simulink model "Uebung5_A1_Anschauungsbeispiel"  (R2016a)
settings: Solver=VariableStepAuto  StartTime=0.0  StopTime=200000  RelTol=1e-3
undefined symbols (not defined in the file or in its folder): m, n
settings Model: Creator=gome  LastModifiedBy=gome

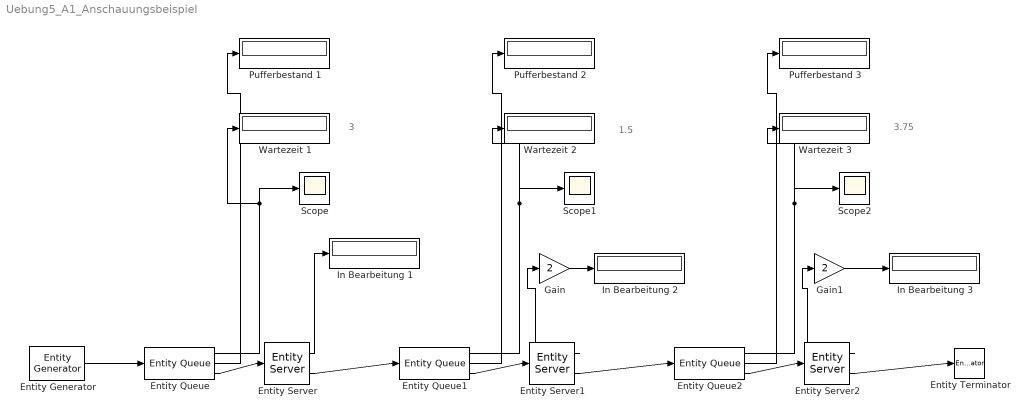
== system Uebung5_A1_Anschauungsbeispiel ==
  note: 3.75
  note: 1.5
  note: 3
  Entity Generator : EntityGenerator  OutputPortMessageModes=m  TimeSource=MATLAB action  IntergenerationTimeAction=|  AttributeName=nextServiceTime  EntityType=Structured  EntityTypeName=Entity
      | persistent init
      | if isempty(init)
      |     init = 1;
      |     rng(235431);
      | end
      | dt = exprnd(1/(336/16/60));
  Entity Queue : EntityQueue  InputPortMessageModes=m  OutputPortMessageModes=n,n,m  Capacity=inf  AverageWait=on  AverageQueueLength=on
      settings: OutputPortMap=o2,o3,o5
  Entity Queue1 : EntityQueue  InputPortMessageModes=m  OutputPortMessageModes=n,n,m  Capacity=inf  PrioritySource=nextServiceTime  AverageWait=on  AverageQueueLength=on
      settings: OutputPortMap=o2,o3,o5
  Entity Queue2 : EntityQueue  InputPortMessageModes=m  OutputPortMessageModes=n,n,m  Capacity=inf  PrioritySource=nextServiceTime  AverageWait=on  AverageQueueLength=on
      settings: OutputPortMap=o2,o3,o5
  Entity Server : EntityServer  InputPortMessageModes=m  OutputPortMessageModes=n,m  Capacity=1  ServiceTimeSource=MATLAB action  ServiceTimeAttributeName=nextServiceTime  ServiceTimeAction=|  Utilization=on
      | persistent init
      | if isempty(init)
      |     init = 1;
      |     rng(3251321);
      | end
      | 
      | m = 2;
      | b = 3.8;
      | dt = m - b/2 + b*rand;
      settings: OutputPortMap=o5,o9
  Entity Server1 : EntityServer  InputPortMessageModes=m  OutputPortMessageModes=n,m  Capacity=2  ServiceTimeSource=MATLAB action  ServiceTimeAttributeName=nextServiceTime  ServiceTimeAction=|  Utilization=on
      | persistent init
      | if isempty(init)
      |     init = 1;
      |     rng(31321);
      | end
      | m = 150/60;
      | dt = 0;
      | p = 0.18;
      | if rand < p
      |     dt = 1/p*m;
      | end
      settings: OutputPortMap=o5,o9
  Entity Server2 : EntityServer  InputPortMessageModes=m  OutputPortMessageModes=n,m  Capacity=2  ServiceTimeSource=MATLAB action  ServiceTimeAttributeName=nextServiceTime  ServiceTimeAction=|  Utilization=on
      | persistent init
      | if isempty(init)
      |     init = 1;
      |     rng(31321);
      | end
      | 
      | m = 135/60;
      | 
      | dt = 0;
      | p = 0.07;
      | if rand < p
      |     dt = 1/p*m;
      | end
      settings: OutputPortMap=o5,o9
  Entity Terminator : EntityTerminator  InputPortMessageModes=m
  Gain : Gain  Gain=2
  Gain1 : Gain  Gain=2
  In Bearbeitung 1 : Display
  In Bearbeitung 2 : Display
  In Bearbeitung 3 : Display
  Pufferbestand 1 : Display
  Pufferbestand 2 : Display
  Pufferbestand 3 : Display
  Scope : Scope
  Scope1 : Scope
  Scope2 : Scope
  Wartezeit 1 : Display
  Wartezeit 2 : Display
  Wartezeit 3 : Display
  wires:
  Entity Generator/1 -> Entity Queue/1
  Entity Server/2 -> Entity Queue1/1
  Entity Server1/2 -> Entity Queue2/1
  Entity Queue/3 -> Entity Server/1
  Entity Queue1/3 -> Entity Server1/1
  Entity Queue2/3 -> Entity Server2/1
  Entity Server2/2 -> Entity Terminator/1
  Entity Queue/1 -> Scope/1, Wartezeit 1/1
  Entity Queue1/1 -> Scope1/1, Wartezeit 2/1
  Entity Queue2/1 -> Scope2/1, Wartezeit 3/1
  Entity Queue2/2 -> Pufferbestand 3/1
  Entity Queue1/2 -> Pufferbestand 2/1
  Entity Queue/2 -> Pufferbestand 1/1
  Entity Server/1 -> In Bearbeitung 1/1
  Gain/1 -> In Bearbeitung 2/1
  Entity Server1/1 -> Gain/1
  Gain1/1 -> In Bearbeitung 3/1
  Entity Server2/1 -> Gain1/1
